simulink model "SIM_CSTR"  (R2023b)
settings: Solver=VariableStepAuto  StartTime=0.0  StopTime=30  RelTol=1e-3
values from neighbouring files (symbols this model uses):
  Ts = 0.05    [MHE_compute.m]    (also in NMPC_CSTR.m)
  u0 = 300    [NMPC_CSTR.m]
libraries: mpclib x1
settings Model: Creator=akeebismail  LastModifiedBy=akeebismail

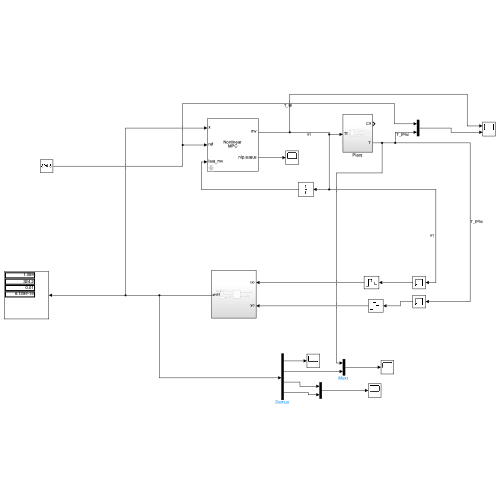
[thumbnail: Simulink's stored preview of the top-level diagram]
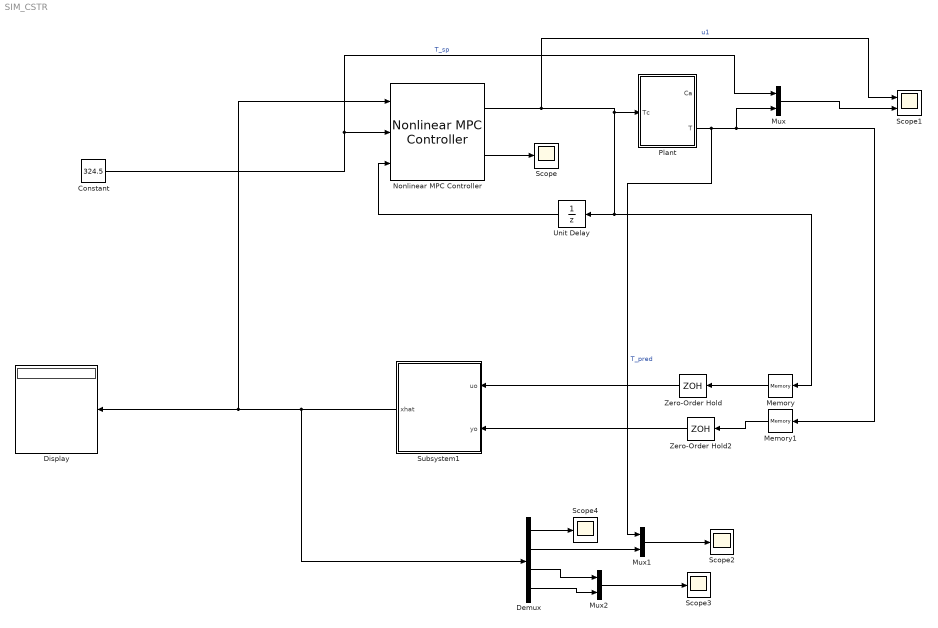
== system SIM_CSTR ==
  Constant : Constant  Value=324.5
  Demux : Demux
  Display : Display
  Memory : Memory  InitialCondition=300
  Memory1 : Memory  InitialCondition=324.5
  Mux : Mux  Inputs=2
  Mux1 : Mux  Inputs=2
  Mux2 : Mux  Inputs=2
  Nonlinear MPC Controller : mpclib/Nonlinear MPC Controller  nlmpcobj=nlobj  UseObjectTs=on  UseMEX=off  md_enabled=off  mvtarget_enabled=off  param_enabled=off  cost_enabled=off  mvseq_enabled=off  stateseq_enabled=off  ovseq_enabled=off  slack_enabled=off  status_enabled=on  ov_min=off  ov_max=off  mv_min=off  mv_max=off  mvrate_min=off  mvrate_max=off  state_min=off  state_max=off  ov_weight=off  mv_weight=off  mvrate_weight=off  ecr_weight=off  nlp_initialize=off
  Plant : Subsystem
  Scope{,2..4} (4 alike) : Scope
  Scope1 : Scope  NumInputPorts=2
  Subsystem1 : Subsystem
  Unit Delay : UnitDelay  InitialCondition=u0  SampleTime=Ts  HasFrameUpgradeWarning=on
  Zero-Order Hold : ZeroOrderHold  SampleTime=Ts
  Zero-Order Hold2 : ZeroOrderHold  SampleTime=Ts
  wires:
  Zero-Order Hold2/1 -> Subsystem1/2(yo)
  Memory/1 -> Zero-Order Hold/1
  Zero-Order Hold/1 -> Subsystem1/1(uo)
  Mux/1 -> Scope1/2
  Memory1/1 -> Zero-Order Hold2/1
  Plant/2(T) -> Mux1/1, Memory1/1, Mux/2  "T_pred"
  Nonlinear MPC Controller/2 -> Scope/1
  Nonlinear MPC Controller/1 -> Scope1/1, Plant/1(Tc), Unit Delay/1, Memory/1  "u1"
  Constant/1 -> Mux/1, Nonlinear MPC Controller/2  "T_sp"
  Unit Delay/1 -> Nonlinear MPC Controller/3
  Subsystem1/1(xhat) -> Demux/1, Nonlinear MPC Controller/1, Display/1
  Demux/2 -> Mux1/2
  Mux1/1 -> Scope2/1
  Demux/3 -> Mux2/1
  Demux/4 -> Mux2/2
  Mux2/1 -> Scope3/1
  Demux/1 -> Scope4/1

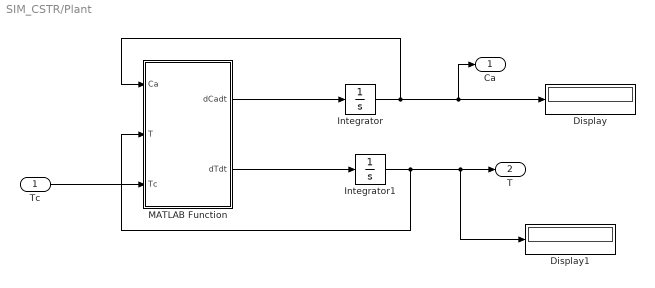
== system SIM_CSTR/Plant ==
  Tc : Inport
  Display : Display
  Display1 : Display
  Integrator : Integrator
  Integrator1 : Integrator  InitialCondition=300
  MATLAB Function : MATLAB Function  TreatAsAtomicUnit=on
  Ca : Outport
  T : Outport  Port=2
  wires:
  Integrator1/1 -> Display1/1, T/1, MATLAB Function/2(T)
  MATLAB Function/2(dTdt) -> Integrator1/1
  Integrator/1 -> Ca/1, Display/1, MATLAB Function/1(Ca)
  MATLAB Function/1(dCadt) -> Integrator/1
  Tc/1 -> MATLAB Function/3(Tc)

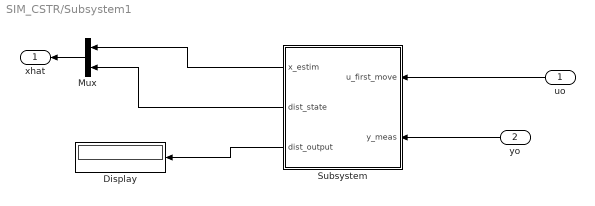
== system SIM_CSTR/Subsystem1 ==
  uo : Inport
  yo : Inport  Port=2
  Display : Display
  Mux : Mux  Inputs=2
  Subsystem : Subsystem
  xhat : Outport
  wires:
  Subsystem/1(x_estim) -> Mux/1
  Subsystem/2(dist_state) -> Mux/2
  Subsystem/3(dist_output) -> Display/1
  uo/1 -> Subsystem/1(u_first_move)
  yo/1 -> Subsystem/2(y_meas)
  Mux/1 -> xhat/1

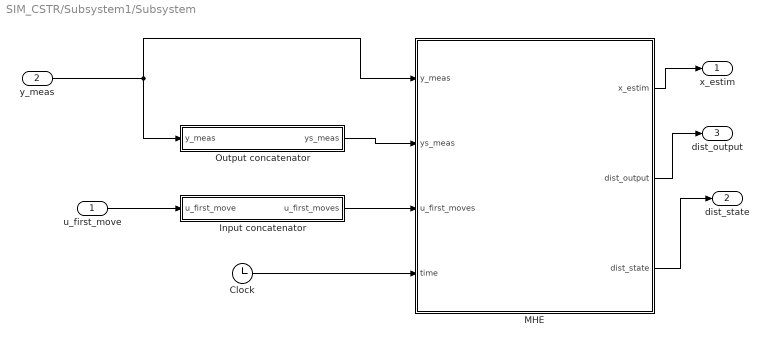
== system SIM_CSTR/Subsystem1/Subsystem ==
  u_first_move : Inport  PortDimensions=[1,1]
  y_meas : Inport  Port=2  PortDimensions=[1,1]
  Clock : Clock
      settings: Decimation=20
  Input concatenator : Subsystem
  MHE : MATLAB Function  TreatAsAtomicUnit=on
  Output concatenator : Subsystem
  x_estim : Outport
  dist_state : Outport  Port=2
  dist_output : Outport  Port=3
  wires:
  Input concatenator/1(u_first_moves) -> MHE/3(u_first_moves)
  MHE/3(dist_state) -> dist_state/1
  MHE/2(dist_output) -> dist_output/1
  Clock/1 -> MHE/4(time)
  u_first_move/1 -> Input concatenator/1(u_first_move)
  MHE/1(x_estim) -> x_estim/1
  y_meas/1 -> MHE/1(y_meas), Output concatenator/1(y_meas)
  Output concatenator/1(ys_meas) -> MHE/2(ys_meas)

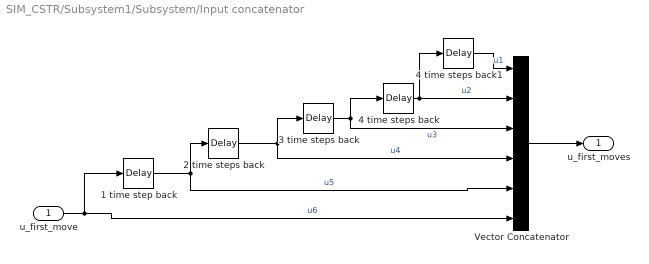
== system SIM_CSTR/Subsystem1/Subsystem/Input concatenator ==
  u_first_move : Inport
  1 time step back : TransportDelay  DelayTime=Ts  InitialOutput=300
  2 time steps back : TransportDelay  DelayTime=Ts  InitialOutput=300
  3 time steps back : TransportDelay  DelayTime=Ts  InitialOutput=300
  4 time steps back : TransportDelay  DelayTime=Ts  InitialOutput=300
  4 time steps back1 : TransportDelay  DelayTime=Ts  InitialOutput=300
  Vector Concatenator : Concatenate  NumInputs=6  Mode=Multidimensional array
  u_first_moves : Outport  PortDimensions=[6,1]  VectorParamsAs1DForOutWhenUnconnected=off
  wires:
  Vector Concatenator/1 -> u_first_moves/1
  u_first_move/1 -> Vector Concatenator/6, 1 time step back/1  "u6"
  4 time steps back/1 -> Vector Concatenator/2, 4 time steps back1/1  "u2"
  3 time steps back/1 -> Vector Concatenator/3, 4 time steps back/1  "u3"
  2 time steps back/1 -> 3 time steps back/1, Vector Concatenator/4  "u4"
  1 time step back/1 -> 2 time steps back/1, Vector Concatenator/5  "u5"
  4 time steps back1/1 -> Vector Concatenator/1  "u1"

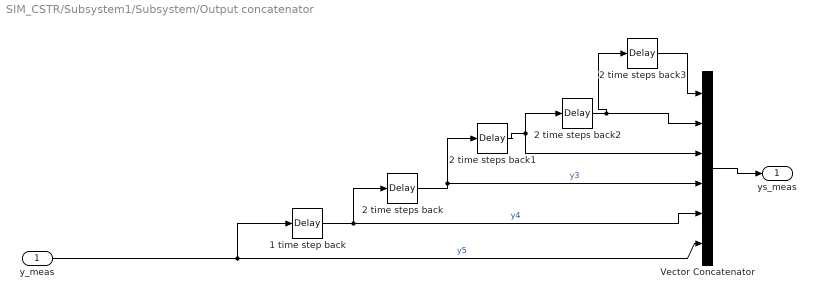
== system SIM_CSTR/Subsystem1/Subsystem/Output concatenator ==
  y_meas : Inport
  1 time step back : TransportDelay  DelayTime=Ts  InitialOutput=324.5
  2 time steps back{,1..3} (4 alike) : TransportDelay  DelayTime=Ts  InitialOutput=324.5
  Vector Concatenator : Concatenate  NumInputs=6  Mode=Multidimensional array
  ys_meas : Outport  PortDimensions=[6,1]  VectorParamsAs1DForOutWhenUnconnected=off
  wires:
  2 time steps back2/1 -> 2 time steps back3/1, Vector Concatenator/2
  2 time steps back1/1 -> 2 time steps back2/1, Vector Concatenator/3
  Vector Concatenator/1 -> ys_meas/1
  2 time steps back/1 -> 2 time steps back1/1, Vector Concatenator/4  "y3"
  1 time step back/1 -> Vector Concatenator/5, 2 time steps back/1  "y4"
  y_meas/1 -> Vector Concatenator/6, 1 time step back/1  "y5"
  2 time steps back3/1 -> Vector Concatenator/1

== matlab function SIM_CSTR/Subsystem1/Subsystem/MHE ==
  data: y_meas input; ys_meas input; x_estim output; u_first_moves input; time input; dist_output output; dist_state output
function [x_estim,dist_output,dist_state] = MHE_4_tanks(y_meas,ys_meas,u_first_moves,time)

coder.extrinsic('MHE_compute');

N_MHE=6;
% Ts=2 ;


if time < 0.3
    
    x_estim =  [0.877;324.5]  ;
   % x_estim = [17;17;17];
    %x_estim = [5.898;1.8];
    dist_state = [0;0];
    dist_output = 0;
else
    
    [x_estim,dist_state,dist_output] = MHE_compute(ys_meas,u_first_moves,N_MHE,y_meas);
    %Note that our horizon must be constant here. It is chosen as 5.
end

end

== matlab function SIM_CSTR/Plant/MATLAB Function ==
  data: Ca input; dCadt output; T input; Tc input; dTdt output
function [dCadt,dTdt] = fcn(Ca,T,Tc)

values = {100,5e4,350,100,1000,0.239,8750,7.2e10,5e4,1};
[F,delta_H,Tf,V,rho,Cp,E_R,k0,U_A,Caf] = values{:};

% Rate constant (Arrhenius equation)
        k = k0 * exp(-E_R / T);
        
        % Mass balance for Ca
        dCadt = F/V * (Caf - Ca) - k * Ca;
        
        % Energy balance for T
        dTdt = F/V * (Tf - T) + (delta_H / (rho * Cp)) * k * Ca + (U_A / (rho * Cp * V)) * (Tc - T);


end
